simulink subsystem "Controler_les_entrees_et_sorties"  (R2020a)
settings: Solver=VariableStepAuto  StartTime=0.0  StopTime=10.0  RelTol=1e-3
model mask{NombreDePiecesMax=10, B=0.1128, r=0.0203, N=66, K_c=1.422}
  mask prompts: NombreDePiecesMax "Nombre de pièces maximal"; B "Magnitude du champ d'induction magnétique (T)"; r "Rayon de la bobine (m)"; N "Nombre de tours de la bobine"; K_c "Gain du capteur de courant"
values from neighbouring files (symbols this model uses):
  f_echant = 22    [default_design_data.mat]    (also in dict.sldd = 22.0)
  K_c = 1.422    [default_design_data.mat]    (also in dict.sldd)
libraries: simulink x1
settings Model: Creator=frfoc1  LastModifiedBy=frfoc1

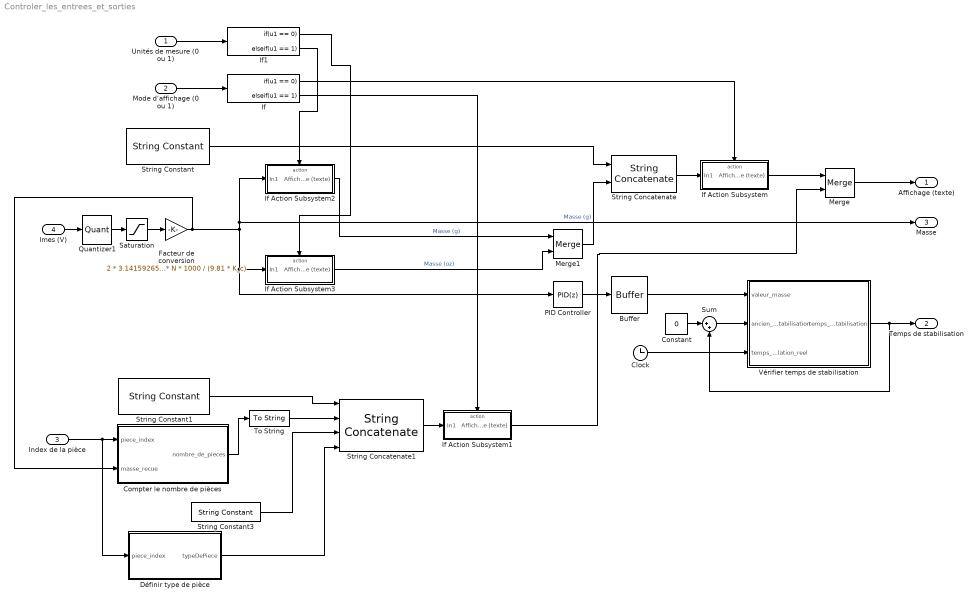
== system Controler_les_entrees_et_sorties ==
  Unités de mesure (0 ou 1) : Inport
  Mode d'affichage (0 ou 1) : Inport  Port=2
  Index de la pièce : Inport  Port=3
  Imes (V) : Inport  Port=4
  Buffer : Buffer  N=10  OutputFrames=off
  Clock : Clock
  Compter le nombre de pièces : MATLAB Function  TreatAsAtomicUnit=on
  Constant : Constant  Value=0
  Définir type de pièce : MATLAB Function  TreatAsAtomicUnit=on
  Facteur de conversion : Gain  Gain=2 * 3.1415926535 * r * B * N * 1000 / (9.81 * K_c)
  If : If  IfExpression=u1 == 0  ElseIfExpressions=u1 == 1  ShowElse=off
  If Action Subsystem : Subsystem  TreatAsAtomicUnit=on
  If Action Subsystem1 : Subsystem  TreatAsAtomicUnit=on
  If Action Subsystem2 : Subsystem  TreatAsAtomicUnit=on
  If Action Subsystem3 : Subsystem  TreatAsAtomicUnit=on
  If1 : If  IfExpression=u1 == 0  ElseIfExpressions=u1 == 1  ShowElse=off
  Merge : Merge
  Merge1 : Merge
  PID Controller : simulink/Continuous/PID Controller  Controller=PID  Form=Parallel  TimeDomain=Discrete-time  UseExternalTs=off  SampleTime=1/f_echant  IntegratorMethod=Forward Euler  FilterMethod=Forward Euler  ControllerParametersSource=internal  P=1  I=0  D=0  UseFilter=on  N=100  TunerSelectOption=Transfer Function Based (PID Tuner App)  InitialConditionSource=internal  InitialConditionForIntegrator=0  InitialConditionForFilter=0  DifferentiatorICPrevScaledInput=0  ExternalReset=none  TrackingMode=off  Kt=1  LimitOutput=off  UpperSaturationLimit=inf  LowerSaturationLimit=-inf  LinearizeAsGain=on  AntiWindupMode=none  Kb=1  POutMin=[]  POutMax=[]  IOutMin=[]  IOutMax=[]  DOutMin=[]  DOutMax=[]  NOutMin=[]  NOutMax=[]  SumOutMin=[]  SumOutMax=[]  SaturationOutMin=[]  SaturationOutMax=[]  PParamMin=[]  PParamMax=[]  IParamMin=[]  IParamMax=[]  DParamMin=[]  DParamMax=[]  NParamMin=[]  NParamMax=[]  KbParamMin=[]  KbParamMax=[]  KtParamMin=[]  KtParamMax=[]  KbOutMin=[]  KbOutMax=[]  KtOutMin=[]  KtOutMax=[]  IntegratorOutMin=[]  IntegratorOutMax=[]  FilterOutMin=[]  FilterOutMax=[]  SumI1OutMin=[]  SumI1OutMax=[]  SumI2OutMin=[]  SumI2OutMax=[]  SumI3OutMin=[]  SumI3OutMax=[]  SumI4OutMin=[]  SumI4OutMax=[]  SumDOutMin=[]  SumDOutMax=[]  DifferentiatorOutMin=[]  DifferentiatorOutMax=[]  FilterDiffOutCoefMin=[]  FilterDiffOutCoefMax=[]  ReciprocalOutMin=[]  ReciprocalOutMax=[]  SumDenOutMin=[]  SumDenOutMax=[]  SumNumOutMin=[]  SumNumOutMax=[]  DivideOutMin=[]  DivideOutMax=[]  UdiffTsProdOutMin=[]  UdiffTsProdOutMax=[]  NTsProdOutMin=[]  NTsProdOutMax=[]  UintegralTsProdOutMin=[]  UintegralTsProdOutMax=[]  UngainTsProdOutMin=[]  UngainTsProdOutMax=[]  IntegratorContinuousStateAttributes=''  IntegratorStateMustResolveToSignalObject=off  IntegratorRTWStateStorageClass=Auto  FilterContinuousStateAttributes=''  FilterStateMustResolveToSignalObject=off  FilterRTWStateStorageClass=Auto  ParallelPVariant=InternalParameters  IdealPVariant=Disabled  IVariant=InternalParameters  DVariant=InternalParameters  IntegratorVariant=Discrete  SatVariant=Disabled  AWVariant=Passthrough  PCopyVariant=Disabled  TRVariant=Disabled  FdbkBlocksVariant=Forward  IdealPFdbkVariant=Disabled  SatFdbkVariant=Disabled  DerivativeFilterVariant=ForwardEulerFilter  NVariant=InternalParameters  NCopyVariant=Disabled  FilterICVariant=InternalICsFilter  IntegratorICVariant=InternalICs  ExternalResetVariant=Disabled  TRSumVariant=Passthrough  SumFdbkVariant=Disabled  SumVariant=Sum_PID  TsampFilterVariant=InternalTs  TsampNgainVariant=Passthrough  TsampIntegralVariant=Passthrough
  Quantizer1 : Quantizer  QuantizationInterval=5/1024  LinearizeAsGain=off
  Saturation : Saturate  UpperLimit=5  LowerLimit=0
  String Concatenate : StringConcatenate
  String Concatenate1 : StringConcatenate  Inputs=4
  String Constant : StringConstant  String="\"Masse totale: \""
  String Constant1 : StringConstant  String="\"Nombre de pièces: \""
  String Constant3 : StringConstant  String="\" x \""
  Sum : Sum  Inputs=|++
  To String : ToString
  Vérifier temps de stabilisation : MATLAB Function  TreatAsAtomicUnit=on
  Affichage (texte) : Outport
  Temps de stabilisation : Outport  Port=2
  Masse : Outport  Port=3
  wires:
  Mode d'affichage (0 ou 1)/1 -> If/1
  Merge/1 -> Affichage (texte)/1
  If Action Subsystem/1(Affichage (texte)) -> Merge/1
  If/2 -> If Action Subsystem1/Action
  If Action Subsystem1/1(Affichage (texte)) -> Merge/2
  If/1 -> If Action Subsystem/Action
  String Constant/1 -> String Concatenate/1
  String Concatenate/1 -> If Action Subsystem/1(In1)
  Unités de mesure (0 ou 1)/1 -> If1/1
  If1/2 -> If Action Subsystem2/Action
  If1/1 -> If Action Subsystem3/Action
  If Action Subsystem3/1(Affichage (texte)) -> Merge1/2  "Masse (oz)"
  If Action Subsystem2/1(Affichage (texte)) -> Merge1/1  "Masse (g)"
  Merge1/1 -> String Concatenate/2
  String Concatenate1/1 -> If Action Subsystem1/1(In1)
  Facteur de conversion/1 -> Masse/1, If Action Subsystem2/1(In1), PID Controller/1, If Action Subsystem3/1(In1), Compter le nombre de pièces/2(masse_recue)  "Masse (g)"
  Index de la pièce/1 -> Compter le nombre de pièces/1(piece_index), Définir type de pièce/1(piece_index)
  String Constant1/1 -> String Concatenate1/1
  Compter le nombre de pièces/1(nombre_de_pieces) -> To String/1
  To String/1 -> String Concatenate1/2
  String Constant3/1 -> String Concatenate1/3
  Définir type de pièce/1(typeDePiece) -> String Concatenate1/4
  Imes (V)/1 -> Quantizer1/1
  Saturation/1 -> Facteur de conversion/1
  Quantizer1/1 -> Saturation/1
  PID Controller/1 -> Buffer/1
  Buffer/1 -> Vérifier temps de stabilisation/1(valeur_masse)
  Vérifier temps de stabilisation/1(temps_de_stabilisation) -> Temps de stabilisation/1, Sum/2
  Sum/1 -> Vérifier temps de stabilisation/2(ancien_temps_de_stabilisation)
  Clock/1 -> Vérifier temps de stabilisation/3(temps_de_simulation_reel)
  Constant/1 -> Sum/1

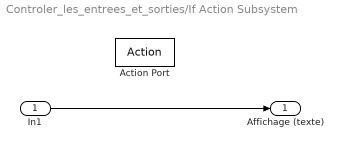
== system Controler_les_entrees_et_sorties/If Action Subsystem ==
  In1 : Inport
  Action Port : ActionPort
  Affichage (texte) : Outport
  wires:
  In1/1 -> Affichage (texte)/1

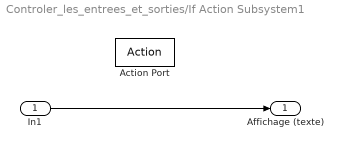
== system Controler_les_entrees_et_sorties/If Action Subsystem1 ==
  In1 : Inport
  Action Port : ActionPort
  Affichage (texte) : Outport
  wires:
  In1/1 -> Affichage (texte)/1

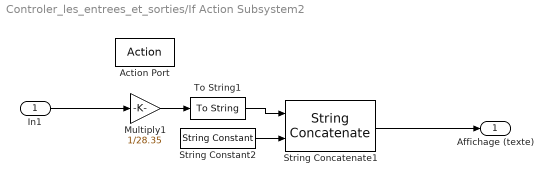
== system Controler_les_entrees_et_sorties/If Action Subsystem2 ==
  In1 : Inport
  Action Port : ActionPort
  Multiply1 : Gain  Gain=1/28.35
  String Concatenate1 : StringConcatenate
  String Constant2 : StringConstant  String="\" oz\""
  To String1 : ToString
  Affichage (texte) : Outport
  wires:
  String Concatenate1/1 -> Affichage (texte)/1
  String Constant2/1 -> String Concatenate1/2
  To String1/1 -> String Concatenate1/1
  Multiply1/1 -> To String1/1
  In1/1 -> Multiply1/1

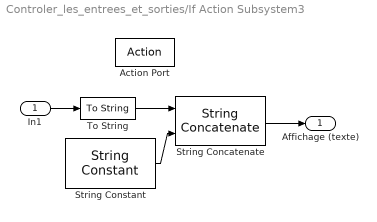
== system Controler_les_entrees_et_sorties/If Action Subsystem3 ==
  In1 : Inport
  Action Port : ActionPort
  String Concatenate : StringConcatenate
  String Constant : StringConstant  String="\" g\""
  To String : ToString
  Affichage (texte) : Outport
  wires:
  String Constant/1 -> String Concatenate/2
  String Concatenate/1 -> Affichage (texte)/1
  To String/1 -> String Concatenate/1
  In1/1 -> To String/1

== matlab function Controler_les_entrees_et_sorties/Définir type de pièce ==
  data: piece_index input; typeDePiece output
function typeDePiece = get_masse_piece(piece_index)
    if piece_index == 0
        typeDePiece = "0.05$"; % 5 cents
    elseif piece_index == 1
        typeDePiece = "0.10$"; % 10 cents
    elseif piece_index == 2
        typeDePiece = "0.25$"; % 25 cents
    elseif piece_index == 3
        typeDePiece = "1.00$"; % 1 dollar
    elseif piece_index == 4
        typeDePiece = "2.00$"; % 2 dollar
    else
        disp("Pièce invalide");
        typeDePiece = "Erreur";
    end

== matlab function Controler_les_entrees_et_sorties/Compter le nombre de pièces ==
  data: piece_index input; nombre_de_pieces output; masse_recue input
function nombre_de_pieces = get_masse_piece(piece_index,masse_recue)
    identificationPieces = [0.05,0.10,0.25,1.00,2.00];
    nombre_de_pieces = 0;
    if piece_index == 0
        masse = 3.950; % 5 cents
    elseif piece_index == 1
        masse = 1.750; % 10 cents
    elseif piece_index == 2
        masse = 4.400; % 25 cents
    elseif piece_index == 3
        masse = 6.270; % 1 dollar
    elseif piece_index == 4
        masse = 6.920; % 2 dollar
    else
        masse = 0;
    end
    dist = inf;
    for x=0:1:10
      if(abs(x*masse - masse_recue) < dist)
        dist = abs(x*masse - masse_recue);
        nombre_de_pieces = x;
      end
    end
    end

== matlab function Controler_les_entrees_et_sorties/Vérifier temps de stabilisation ==
  data: valeur_masse input; temps_de_stabilisation output; ancien_temps_de_stabilisation input; temps_de_simulation_reel input
function temps_de_stabilisation = get_temps_stabilisation(valeur_masse,ancien_temps_de_stabilisation,temps_de_simulation_reel)
    isStable = true;
    margeDeStabilite = 0.03;
    for n = 1: length(valeur_masse) - 1
        for i = n+1: length(valeur_masse)
            if (valeur_masse(n)/valeur_masse(i) <= 1 - margeDeStabilite || 1 + margeDeStabilite <= valeur_masse(n)/valeur_masse(i))
                isStable = false;
            end
        end
    end
    if (isStable == false)
        temps_de_stabilisation = temps_de_simulation_reel;
    else
        temps_de_stabilisation = ancien_temps_de_stabilisation;
    end
end
